simulink model "pendulum_simple"  (R2015b)
settings: Solver=ode4  StartTime=0.0  StopTime=10  FixedStep=1e-3  RelTol=1e-3
values from neighbouring files (symbols this model uses):
  g = 9.8    [pendulum_simple_ilqr.m]    (also in pendulum_simple_ilqr_ddp_derivation.m = zeros(n,N); pendulum_simple_ilqr_my_derivation.m; pendulum_simple_run.m)
  l = 1    [pendulum_simple_ilqr.m]    (also in pendulum_simple_ilqr_ddp_derivation.m; pendulum_simple_ilqr_my_derivation.m; pendulum_simple_run.m)
  m = 1    [pendulum_simple_ilqr.m]    (also in pendulum_simple_ilqr_ddp_derivation.m; pendulum_simple_ilqr_my_derivation.m; pendulum_simple_run.m)
  mu = 0.01    [pendulum_simple_ilqr.m]    (also in pendulum_simple_ilqr_ddp_derivation.m; pendulum_simple_ilqr_my_derivation.m; pendulum_simple_run.m)
  theta0 = pi/2    (= 1.57079632679)    [pendulum_simple_run.m]
  thetad0 = 0    [pendulum_simple_run.m]
settings Model: Creator=taylor howell  LastModifiedBy=taylor howell

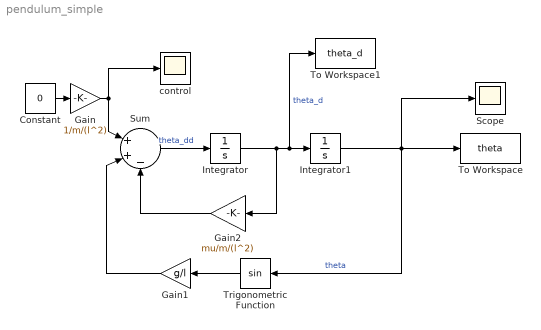
== system pendulum_simple ==
  Constant : Constant  Value=0
  Gain : Gain  Gain=1/m/(l^2)
  Gain1 : Gain  Gain=g/l
  Gain2 : Gain  Gain=mu/m/(l^2)
  Integrator : Integrator  InitialCondition=thetad0
  Integrator1 : Integrator  InitialCondition=theta0
  Scope : Scope
  Sum : Sum  Inputs=|++-
  To Workspace : ToWorkspace  VariableName=theta  SaveFormat=Timeseries  SampleTime=-1
  To Workspace1 : ToWorkspace  VariableName=theta_d  SaveFormat=Timeseries  SampleTime=-1
  Trigonometric Function : Trigonometry
  control : Scope
  wires:
  Integrator/1 -> Gain2/1, To Workspace1/1, Integrator1/1  "theta_d"
  Integrator1/1 -> Scope/1, To Workspace/1, Trigonometric Function/1  "theta"
  Gain2/1 -> Sum/3
  Gain/1 -> Sum/1, control/1
  Trigonometric Function/1 -> Gain1/1
  Gain1/1 -> Sum/2
  Sum/1 -> Integrator/1  "theta_dd"
  Constant/1 -> Gain/1
